simulink model "Final_Assem2_temp"  (R2021b)
settings: Solver=VariableStepAuto  StartTime=0.0  StopTime=10  RelTol=1e-3
model workspace: external: MATLAB File D:\university\Semester 8\Intro to Robotics\Project\amali\Final_3\export second\Final_Assem_DataFile.m (data not in the file)
settings Model: Creator=admin  LastModifiedBy=ASUS

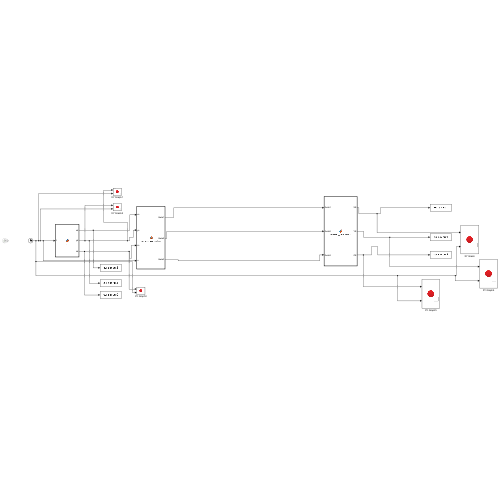
[thumbnail: Simulink's stored preview of the top-level diagram]
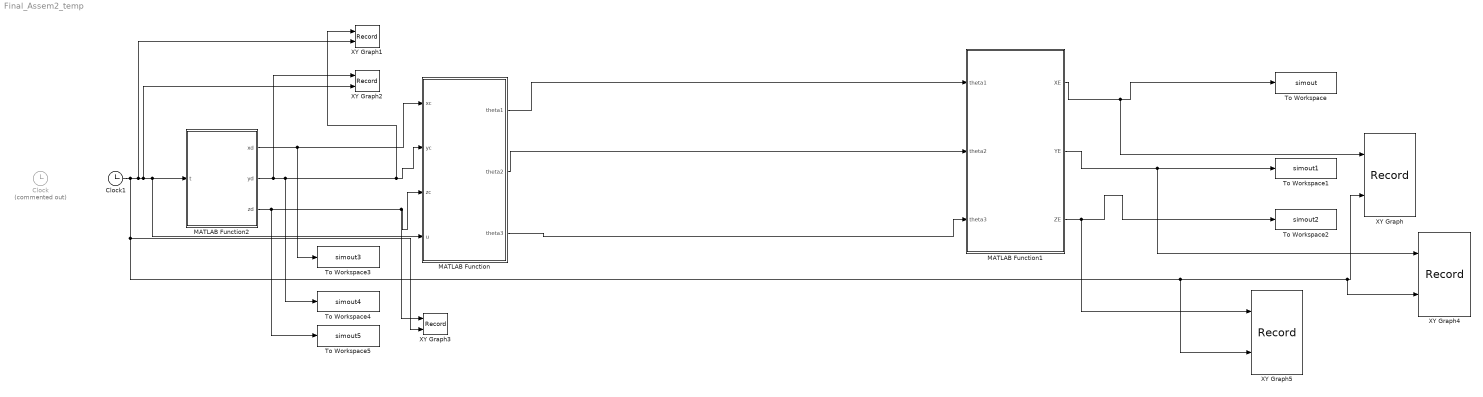
== system Final_Assem2_temp ==
  Clock : Clock  Commented=on
      settings: Decimation=u
  Clock1 : Clock
  MATLAB Function : MATLAB Function  TreatAsAtomicUnit=on
  MATLAB Function1 : MATLAB Function  TreatAsAtomicUnit=on
  MATLAB Function2 : MATLAB Function  TreatAsAtomicUnit=on
  To Workspace : ToWorkspace  VariableName=simout  SampleTime=-1
      settings: Save2DSignal=2-D array (concatenate along first dimension)
  To Workspace1 : ToWorkspace  VariableName=simout1  SampleTime=-1
      settings: Save2DSignal=2-D array (concatenate along first dimension)
  To Workspace2 : ToWorkspace  VariableName=simout2  SampleTime=-1
      settings: Save2DSignal=2-D array (concatenate along first dimension)
  To Workspace3 : ToWorkspace  VariableName=simout3  SampleTime=-1
      settings: Save2DSignal=2-D array (concatenate along first dimension)
  To Workspace4 : ToWorkspace  VariableName=simout4  SampleTime=-1
      settings: Save2DSignal=2-D array (concatenate along first dimension)
  To Workspace5 : ToWorkspace  VariableName=simout5  SampleTime=-1
      settings: Save2DSignal=2-D array (concatenate along first dimension)
  XY Graph : Record  FileSettingsInternal="{\"entries\":[{\"content\":{\"excelSettings\":{\"content\":{},\"type\":\"Streamout.ExcelSettings\"}},\"type\":\"Streamout.FileSettingStorage\",\"uuid\":\"4b2bbe7e-8042-4974-99ab-08a61305e2c4\"}],\"packageUris\":[\"http://schema.mathworks.com/mf0/streamout_blocks/R2020a\"],\"version\":\"1.0\"}"  Layout=[1 1]  SignalsInternal="{\"entries\":[{\"content\":{\"signals\":[{\"content\":{\"blockPath\":[\"Final_Assem2_temp/XY Graph\"],\"channel\":[],\"dimensions\":[1],\"domain\":\"Final_Assem2_temp/XY Graph\",\"lineColor\":\"#a2142f\",\"plots\":[1],\"port\":1,\"sid\":[\"\"],\"signalID\":1927,\"signalName\":\"MATLAB Function1:1\"},\"type\":\"RecordBlkView.Signal\",\"uuid\":\"c76d3085-ffb2-4c06-b09b-2b35fb36873a\"},{\"content\":{\"blockPath\":[\"Final_Assem2_temp/XY Graph\"],\"channel\":[],\"dimensions\":[1],\"domain\":\"Final_Assem2_temp/XY Graph\",\"lineColor\":\"#139fff\",\"plots\":[1],\"port\":2,\"sid\":[\"\"],\"signalID\":1931,\"signalName\":\"Clock1\"},\"type\":\"RecordBlkView.Signal\",\"uuid\":\"d9713151-38d3-4a94-9135-5ec86b9d4622\"}]},\"type\":\"RecordBlkView.InputSignals\",\"uuid\":\"2bdd9db9-c01a-4d06-b307-77267f663fc6\"}],\"packageUris\":[\"http://schema.mathworks.com/mf0/streamout_blocks/R2020a\"],\"version\":\"1.0\"}"  VisualizationBindings="{\"xyplotplugin\":{\"info\":[{\"series\":[{\"bindingParametersList\":[{\"parameter\":\"X-Axis\",\"signalID\":1927,\"signalName\":\"MATLAB Function1:1\"},{\"parameter\":\"Y-Axis\",\"signalID\":1931,\"signalName\":\"Clock1\"}],\"seriesID\":54939}],\"subplotID\":1}]}}"  CompatibilityTag=XY
  XY Graph1 : Record  FileSettingsInternal="{\"entries\":[{\"content\":{\"excelSettings\":{\"content\":{},\"type\":\"Streamout.ExcelSettings\"}},\"type\":\"Streamout.FileSettingStorage\",\"uuid\":\"50392818-c749-4776-a8d3-2162c3cfa793\"}],\"packageUris\":[\"http://schema.mathworks.com/mf0/streamout_blocks/R2020a\"],\"version\":\"1.0\"}"  Layout=[1 1]  SignalsInternal="{\"entries\":[{\"content\":{\"signals\":[{\"content\":{\"blockPath\":[\"Final_Assem2_temp/XY Graph1\"],\"channel\":[],\"dimensions\":[1],\"domain\":\"Final_Assem2_temp/XY Graph1\",\"lineColor\":\"#a2142f\",\"plots\":[1],\"port\":1,\"sid\":[\"\"],\"signalID\":1935,\"signalName\":\"MATLAB Function2:2\"},\"type\":\"RecordBlkView.Signal\",\"uuid\":\"1623001a-22c0-4cb0-a8e9-beb7106a292c\"},{\"content\":{\"blockPath\":[\"Final_Assem2_temp/XY Graph1\"],\"channel\":[],\"dimensions\":[1],\"domain\":\"Final_Assem2_temp/XY Graph1\",\"lineColor\":\"#139fff\",\"plots\":[1],\"port\":2,\"sid\":[\"\"],\"signalID\":1939,\"signalName\":\"Clock1\"},\"type\":\"RecordBlkView.Signal\",\"uuid\":\"f4ec799c-8b5e-4fd7-aeb1-64109254df47\"}]},\"type\":\"RecordBlkView.InputSignals\",\"uuid\":\"ea3f0653-04e0-48aa-943b-a3e63e2f143b\"}],\"packageUris\":[\"http://schema.mathworks.com/mf0/streamout_blocks/R2020a\"],\"version\":\"1.0\"}"  VisualizationBindings="{\"xyplotplugin\":{\"info\":[{\"series\":[{\"bindingParametersList\":[{\"parameter\":\"X-Axis\",\"signalID\":1935,\"signalName\":\"MATLAB Function2:2\"},{\"parameter\":\"Y-Axis\",\"signalID\":1939,\"signalName\":\"Clock1\"}],\"seriesID\":28193}],\"subplotID\":1}]}}"  CompatibilityTag=XY
  XY Graph2 : Record  FileSettingsInternal="{\"entries\":[{\"content\":{\"excelSettings\":{\"content\":{},\"type\":\"Streamout.ExcelSettings\"}},\"type\":\"Streamout.FileSettingStorage\",\"uuid\":\"3fc0da13-8ce4-4b04-bb40-563668f06fb2\"}],\"packageUris\":[\"http://schema.mathworks.com/mf0/streamout_blocks/R2020a\"],\"version\":\"1.0\"}"  Layout=[1 1]  SignalsInternal="{\"entries\":[{\"content\":{\"signals\":[{\"content\":{\"blockPath\":[\"Final_Assem2_temp/XY Graph2\"],\"channel\":[],\"dimensions\":[1],\"domain\":\"Final_Assem2_temp/XY Graph2\",\"lineColor\":\"#a2142f\",\"plots\":[1],\"port\":1,\"sid\":[\"\"],\"signalID\":1943,\"signalName\":\"MATLAB Function2:2\"},\"type\":\"RecordBlkView.Signal\",\"uuid\":\"6afcc2c0-6dad-4f7a-80d9-79bee599c8ff\"},{\"content\":{\"blockPath\":[\"Final_Assem2_temp/XY Graph2\"],\"channel\":[],\"dimensions\":[1],\"domain\":\"Final_Assem2_temp/XY Graph2\",\"lineColor\":\"#139fff\",\"plots\":[1],\"port\":2,\"sid\":[\"\"],\"signalID\":1947,\"signalName\":\"Clock1\"},\"type\":\"RecordBlkView.Signal\",\"uuid\":\"dd6633d8-a05d-4c6e-ae3c-7299fff014d9\"}]},\"type\":\"RecordBlkView.InputSignals\",\"uuid\":\"4df68c6c-9f24-4879-b23e-10f6ca3217f7\"}],\"packageUris\":[\"http://schema.mathworks.com/mf0/streamout_blocks/R2020a\"],\"version\":\"1.0\"}"  VisualizationBindings="{\"xyplotplugin\":{\"info\":[{\"series\":[{\"bindingParametersList\":[{\"parameter\":\"X-Axis\",\"signalID\":1943,\"signalName\":\"MATLAB Function2:2\"},{\"parameter\":\"Y-Axis\",\"signalID\":1947,\"signalName\":\"Clock1\"}],\"seriesID\":47343}],\"subplotID\":1}]}}"  CompatibilityTag=XY
  XY Graph3 : Record  FileSettingsInternal="{\"entries\":[{\"content\":{\"excelSettings\":{\"content\":{},\"type\":\"Streamout.ExcelSettings\"}},\"type\":\"Streamout.FileSettingStorage\",\"uuid\":\"923f3d11-ab1e-4f43-a458-d864e7b86e82\"}],\"packageUris\":[\"http://schema.mathworks.com/mf0/streamout_blocks/R2020a\"],\"version\":\"1.0\"}"  Layout=[1 1]  SignalsInternal="{\"entries\":[{\"content\":{\"signals\":[{\"content\":{\"blockPath\":[\"Final_Assem2_temp/XY Graph3\"],\"channel\":[],\"dimensions\":[1],\"domain\":\"Final_Assem2_temp/XY Graph3\",\"lineColor\":\"#a2142f\",\"plots\":[1],\"port\":1,\"sid\":[\"\"],\"signalID\":1951,\"signalName\":\"MATLAB Function2:3\"},\"type\":\"RecordBlkView.Signal\",\"uuid\":\"0b488fd0-09ee-4480-87b0-cc211f7d6cd7\"},{\"content\":{\"blockPath\":[\"Final_Assem2_temp/XY Graph3\"],\"channel\":[],\"dimensions\":[1],\"domain\":\"Final_Assem2_temp/XY Graph3\",\"lineColor\":\"#139fff\",\"plots\":[1],\"port\":2,\"sid\":[\"\"],\"signalID\":1955,\"signalName\":\"Clock1\"},\"type\":\"RecordBlkView.Signal\",\"uuid\":\"7a06c176-bc7e-4619-bbce-771d1c44eea2\"}]},\"type\":\"RecordBlkView.InputSignals\",\"uuid\":\"6b24e960-d695-4a27-b748-a6c6452fed8c\"}],\"packageUris\":[\"http://schema.mathworks.com/mf0/streamout_blocks/R2020a\"],\"version\":\"1.0\"}"  VisualizationBindings="{\"xyplotplugin\":{\"info\":[{\"series\":[{\"bindingParametersList\":[{\"parameter\":\"X-Axis\",\"signalID\":1951,\"signalName\":\"MATLAB Function2:3\"},{\"parameter\":\"Y-Axis\",\"signalID\":1955,\"signalName\":\"Clock1\"}],\"seriesID\":14445}],\"subplotID\":1}]}}"  CompatibilityTag=XY
  XY Graph4 : Record  FileSettingsInternal="{\"entries\":[{\"content\":{\"excelSettings\":{\"content\":{},\"type\":\"Streamout.ExcelSettings\"}},\"type\":\"Streamout.FileSettingStorage\",\"uuid\":\"668417a1-cfa6-40b5-8bac-8834a77931f6\"}],\"packageUris\":[\"http://schema.mathworks.com/mf0/streamout_blocks/R2020a\"],\"version\":\"1.0\"}"  Layout=[1 1]  SignalsInternal="{\"entries\":[{\"content\":{\"signals\":[{\"content\":{\"blockPath\":[\"Final_Assem2_temp/XY Graph4\"],\"channel\":[],\"dimensions\":[1],\"domain\":\"Final_Assem2_temp/XY Graph4\",\"lineColor\":\"#a2142f\",\"plots\":[1],\"port\":1,\"sid\":[\"\"],\"signalID\":1959,\"signalName\":\"MATLAB Function1:2\"},\"type\":\"RecordBlkView.Signal\",\"uuid\":\"60fbb069-cc66-4adc-b353-845a086bdcdf\"},{\"content\":{\"blockPath\":[\"Final_Assem2_temp/XY Graph4\"],\"channel\":[],\"dimensions\":[1],\"domain\":\"Final_Assem2_temp/XY Graph4\",\"lineColor\":\"#139fff\",\"plots\":[1],\"port\":2,\"sid\":[\"\"],\"signalID\":1963,\"signalName\":\"Clock1\"},\"type\":\"RecordBlkView.Signal\",\"uuid\":\"cada1dc9-dc37-4587-977d-29f8307f942e\"}]},\"type\":\"RecordBlkView.InputSignals\",\"uuid\":\"45e2d337-d591-446a-9402-52f20b196381\"}],\"packageUris\":[\"http://schema.mathworks.com/mf0/streamout_blocks/R2020a\"],\"version\":\"1.0\"}"  VisualizationBindings="{\"xyplotplugin\":{\"info\":[{\"series\":[{\"bindingParametersList\":[{\"parameter\":\"X-Axis\",\"signalID\":1959,\"signalName\":\"MATLAB Function1:2\"},{\"parameter\":\"Y-Axis\",\"signalID\":1963,\"signalName\":\"Clock1\"}],\"seriesID\":63824}],\"subplotID\":1}]}}"  CompatibilityTag=XY
  XY Graph5 : Record  FileSettingsInternal="{\"entries\":[{\"content\":{\"excelSettings\":{\"content\":{},\"type\":\"Streamout.ExcelSettings\"}},\"type\":\"Streamout.FileSettingStorage\",\"uuid\":\"19749252-13f8-4166-b0dd-996ca3f10f9e\"}],\"packageUris\":[\"http://schema.mathworks.com/mf0/streamout_blocks/R2020a\"],\"version\":\"1.0\"}"  Layout=[1 1]  SignalsInternal="{\"entries\":[{\"content\":{\"signals\":[{\"content\":{\"blockPath\":[\"Final_Assem2_temp/XY Graph5\"],\"channel\":[],\"dimensions\":[1],\"domain\":\"Final_Assem2_temp/XY Graph5\",\"lineColor\":\"#a2142f\",\"plots\":[1],\"port\":1,\"sid\":[\"\"],\"signalID\":1967,\"signalName\":\"MATLAB Function1:3\"},\"type\":\"RecordBlkView.Signal\",\"uuid\":\"f523291a-61b9-45c5-a7b2-06bdbcdd2877\"},{\"content\":{\"blockPath\":[\"Final_Assem2_temp/XY Graph5\"],\"channel\":[],\"dimensions\":[1],\"domain\":\"Final_Assem2_temp/XY Graph5\",\"lineColor\":\"#139fff\",\"plots\":[1],\"port\":2,\"sid\":[\"\"],\"signalID\":1971,\"signalName\":\"Clock1\"},\"type\":\"RecordBlkView.Signal\",\"uuid\":\"b2fc1e6e-4534-48b5-ba66-32ba0971a348\"}]},\"type\":\"RecordBlkView.InputSignals\",\"uuid\":\"5dadb43e-634e-4cc0-9820-246fcdac9764\"}],\"packageUris\":[\"http://schema.mathworks.com/mf0/streamout_blocks/R2020a\"],\"version\":\"1.0\"}"  VisualizationBindings="{\"xyplotplugin\":{\"info\":[{\"series\":[{\"bindingParametersList\":[{\"parameter\":\"X-Axis\",\"signalID\":1967,\"signalName\":\"MATLAB Function1:3\"},{\"parameter\":\"Y-Axis\",\"signalID\":1971,\"signalName\":\"Clock1\"}],\"seriesID\":36171}],\"subplotID\":1}]}}"  CompatibilityTag=XY
  wires:
  MATLAB Function2/1(xd) -> To Workspace3/1, MATLAB Function/1(xc)
  MATLAB Function2/2(yd) -> XY Graph2/1, To Workspace4/1, XY Graph1/1, MATLAB Function/2(yc)
  MATLAB Function2/3(zd) -> To Workspace5/1, XY Graph3/1, MATLAB Function/3(zc)
  MATLAB Function/2(theta2) -> MATLAB Function1/2(theta2)
  MATLAB Function/1(theta1) -> MATLAB Function1/1(theta1)
  MATLAB Function/3(theta3) -> MATLAB Function1/3(theta3)
  MATLAB Function1/1(XE) -> XY Graph/1, To Workspace/1
  MATLAB Function1/2(YE) -> XY Graph4/1, To Workspace1/1
  MATLAB Function1/3(ZE) -> XY Graph5/1, To Workspace2/1
  Clock1/1 -> XY Graph3/2, XY Graph5/2, XY Graph4/2, XY Graph/2, XY Graph1/2, XY Graph2/2, MATLAB Function/4(u), MATLAB Function2/1(t)

== matlab function Final_Assem2_temp/MATLAB Function1 ==
  data: theta1 input; XE output; theta2 input; theta3 input; YE output; ZE output
function [XE,YE,ZE]= forward_kinematics(theta1,theta2,theta3)
% 
% 
% xa= 0.224*cos(theta1)*sin(theta2) - 0.06821*cos(theta1) + 0.1*cos(theta1)*cos(theta2)*sin(theta3) + 0.1*cos(theta1)*cos(theta3)*sin(theta2);
% ya= 0.224*cos(theta1)*sin(theta2) - 0.06821*cos(theta1) + 0.1*cos(theta1)*cos(theta2)*sin(theta3) + 0.1*cos(theta1)*cos(theta3)*sin(theta2);
% za= 0.1*cos(theta2 + theta3) + 0.224*cos(theta2) + 0.178;

%a
a1=0;
a2=-0.06821;
a3=0.224;
a4 = 0;
%alpha
alphab1=  0;
alphab2= -pi/2;
alphab3=  0;
alphab4= -pi/2;
% d
d1 = 0.178;
d2 = 0;
d3 = 0;
d4 = 0.1;
%theta
theta2 = -pi/2 + theta2;
theta3 = -pi/2 + theta3;
theta4 = 0;
T1=[cos(theta1) -sin(theta1) 0 a1;
   sin(theta1)*cos(alphab1) cos(theta1)*cos(alphab1) -sin(alphab1) -sin(alphab1)*d1;
   sin(theta1)*sin(alphab1) cos(theta1)*sin(alphab1) cos(alphab1) cos(alphab1)*d1;
   0 0 0 1];
T2=[cos(theta2) -sin(theta2) 0 a2;
   sin(theta2)*cos(alphab2) cos(theta2)*cos(alphab2) -sin(alphab2) -sin(alphab2)*d2;
   sin(theta2)*sin(alphab2) cos(theta2)*sin(alphab2) cos(alphab2) cos(alphab2)*d2;
   0 0 0 1];
T3=[cos(theta3) -sin(theta3) 0 a3;
   sin(theta3)*cos(alphab3) cos(theta3)*cos(alphab3) -sin(alphab3) -sin(alphab3)*d3;
   sin(theta3)*sin(alphab3) cos(theta3)*sin(alphab3) cos(alphab3) cos(alphab3)*d3;
   0 0 0 1];
 T4=[cos(theta4) -sin(theta4) 0 a4;
    sin(theta4)*cos(alphab4) cos(theta4)*cos(alphab4) -sin(alphab4) -sin(alphab4)*d4;
   sin(theta4)*sin(alphab4) cos(theta4)*sin(alphab4) cos(alphab4) cos(alphab4)*d4;
    0 0 0 1];
Ttotal = T1*T2*T3*T4;
XE = Ttotal(1,4);
YE = Ttotal(2,4);
ZE = Ttotal(3,4);

== matlab function Final_Assem2_temp/MATLAB Function ==
  data: xc input; theta1 output; yc input; zc input; theta2 output; theta3 output; u input
function [theta1,theta2,theta3]= inverse_kinematics(xc,yc,zc,u)
theta1 = atan2(yc,xc)

xprim = (xc /cos(theta1))+ 0.0682;
yprim = (yc /sin(theta1))+0.0682;
zprim = zc - 0.178;
c_3 = (yprim^2+zprim^2-0.06)/(0.0449);
s_3 =(1-(1/2)*c_3^2);
theta3 = atan2(s_3,c_3)

c_2=((0.224*cos(theta1)+0.1*cos(theta3)*cos(theta1))*(zc-0.178))-(0.1*cos(theta3)*(xc+0.0682));
s_2=((xc+0.0682)*(0.1*sin(theta3)+0.224))-(zc-0.178)*(0.1*sin(theta3)*cos(theta1));
theta2 = atan2(s_2,c_2)
% d= 0.0165;
% d1= 0.196;
% a2= 0.217;
% a3=0.1;
% phi= atan2(xc,yc);
% r=sqrt(xc^2+yc^2);
% alpha= atan2(sqrt(r^2-d^2),d);
% theta1= phi- alpha
% s= zc-d1;
% rprim= sqrt(xc^2+yc^2-d^2);
% D= (rprim^2+s^2 - a2^2 - a3^2)/(2*a2*a3);
% if(u<5)
% theta3= atan2(D,sqrt(abs(1-D^2)))
% theta2=atan2(rprim,s)- atan2(a2 + a3*cos(theta3),a3*sin(theta3))
% else
% theta3= atan2(D,-sqrt(abs(1-D^2)));
% theta2=atan2(rprim,s)- atan2(a2 + a3*cos(theta3),a3*sin(theta3))
% end

== matlab function Final_Assem2_temp/MATLAB Function2 ==
  data: t input; xd output; yd output; zd output
function [xd,yd,zd]=DT(t)

% xd= 0.2 - 0.2*sin((2*pi/5)*u + pi/2);
% yd= 0.3; %-1 - 0.5*cos((2*pi/5)*u + pi/2);
% zd= -0.5 - 0.5*cos((2*pi/5)*u + pi/2);
if(t<5)
x0=0.2;
y0=0.07; %0.1
z0=0;
x1=-0.1;
y1=0;
z1=0.25;
s=t/5;
xd=x0+(x1-x0)*s; 
yd=y0+(y1-y0)*s;
zd=z0+(z1-z0)*s;
else
x0=-0.1;
y0=0; %0.1
z0=0.25;
x1=0.2;
y1=0.07;
z1=0;
s=(t-5)/5;
xd=x0+(x1-x0)*s; 
yd=y0+(y1-y0)*s;
zd=z0+(z1-z0)*s;
end
